simulink model "momentumBasedFlight"  (R2023b)
settings: Solver=VariableStepAuto  StartTime=0.0  StopTime=Config.simulationTime  RelTol=1e-3
InitFcn:
  | cd(fileparts(which(bdroot)));
  | initMomentumBasedFlight;
StopFcn:
  | cd(fileparts(which(bdroot)));
  | stopMomentumBasedFlight;
undefined symbols (not defined in the file or in its folder): aero_config, biasVectorConstraint_feet, Config, confVisualizer, ConstraintMatrix_feet, DiscIntNeverNeededParam, frameNames, Frames, jets_config, robot_config
libraries: WBToolboxLibrary x82, momentum_flight_control_v1 x1, deeplib x1, mwbs_robotDynamicsWithContacts_lib x1
(part 2 of 3)

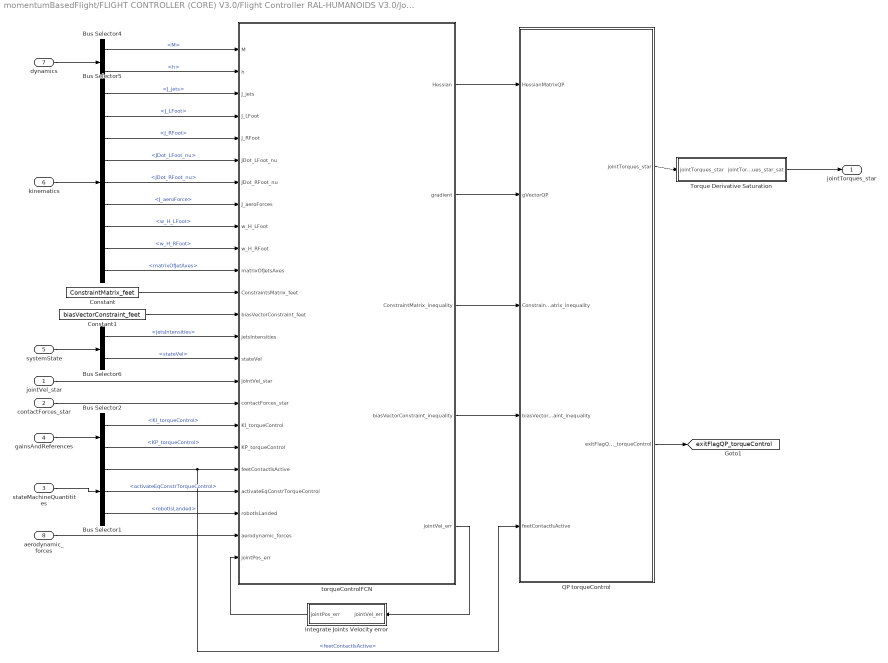
== system momentumBasedFlight/FLIGHT CONTROLLER (CORE) V3.0/Flight Controller RAL-HUMANOIDS V3.0/Joint Torque Control for Flying ==
  jointVel_star : Inport
  contactForces_star : Inport  Port=2
  stateMachineQuantitites : Inport  Port=3
  gainsAndReferences : Inport  Port=4
  systemState : Inport  Port=5
  kinematics : Inport  Port=6
  dynamics : Inport  Port=7
  aerodynamic_forces : Inport  Port=8
  Bus Selector1 : BusSelector  OutputSignals=feetContactIsActive,activateEqConstrTorqueControl,robotIsLanded
  Bus Selector2 : BusSelector  OutputSignals=KI_torqueControl,KP_torqueControl
  Bus Selector4 : BusSelector  OutputSignals=M,h
  Bus Selector5 : BusSelector  OutputSignals=J_jets,J_LFoot,J_RFoot,JDot_LFoot_nu,JDot_RFoot_nu,J_aeroForce,w_H_LFoot,w_H_RFoot,matrixOfJetAxes
  Bus Selector6 : BusSelector  OutputSignals=jetsIntensities,stateVel
  Constant : Constant  Value=ConstraintMatrix_feet
  Constant1 : Constant  Value=biasVectorConstraint_feet
  Integrate Joints Velocity error : Subsystem
  QP torqueControl : Subsystem
  Torque Derivative Saturation : Subsystem
  torqueControlFCN : MATLAB Function  TreatAsAtomicUnit=on
  jointTorques_star : Outport  VectorParamsAs1DForOutWhenUnconnected=off
  tag scope: exitFlagQP_torqueControl=global
  wires:
  Torque Derivative Saturation/1(jointTorques_star_sat) -> jointTorques_star/1
  Bus Selector1/2 -> torqueControlFCN/21(activateEqConstrTorqueControl)  "<activateEqConstrTorqueControl>"
  Bus Selector1/3 -> torqueControlFCN/22(robotIsLanded)  "<robotIsLanded>"
  torqueControlFCN/5(jointVel_err) -> Integrate Joints Velocity error/1(jointVel_err)
  Integrate Joints Velocity error/1(jointPos_err) -> torqueControlFCN/24(jointPos_err)
  Bus Selector5/9 -> torqueControlFCN/11(matrixOfJetsAxes)  "<matrixOfJetAxes>"
  jointVel_star/1 -> torqueControlFCN/16(jointVel_star)
  torqueControlFCN/4(biasVectorConstraint_inequality) -> QP torqueControl/4(biasVectorConstraint_inequality)
  torqueControlFCN/3(ConstraintMatrix_inequality) -> QP torqueControl/3(ConstraintMatrix_inequality)
  torqueControlFCN/2(gradient) -> QP torqueControl/2(gVectorQP)
  torqueControlFCN/1(Hessian) -> QP torqueControl/1(HessianMatrixQP)
  Bus Selector2/2 -> torqueControlFCN/19(KP_torqueControl)  "<KP_torqueControl>"
  Bus Selector2/1 -> torqueControlFCN/18(KI_torqueControl)  "<KI_torqueControl>"
  gainsAndReferences/1 -> Bus Selector2/1
  Bus Selector1/1 -> QP torqueControl/5(feetContactIsActive), torqueControlFCN/20(feetContactIsActive)  "<feetContactIsActive>"
  stateMachineQuantitites/1 -> Bus Selector1/1
  Bus Selector6/1 -> torqueControlFCN/14(jetsIntensities)  "<jetsIntensities>"
  QP torqueControl/2(exitFlagQP_torqueControl) -> [exitFlagQP_torqueControl]
  QP torqueControl/1(jointTorques_star) -> Torque Derivative Saturation/1(jointTorques_star)
  contactForces_star/1 -> torqueControlFCN/17(contactForces_star)
  Constant/1 -> torqueControlFCN/12(ConstraintsMatrix_feet)
  Constant1/1 -> torqueControlFCN/13(biasVectorConstraint_feet)
  Bus Selector5/8 -> torqueControlFCN/10(w_H_RFoot)  "<w_H_RFoot>"
  Bus Selector5/7 -> torqueControlFCN/9(w_H_LFoot)  "<w_H_LFoot>"
  Bus Selector5/5 -> torqueControlFCN/7(JDot_RFoot_nu)  "<JDot_RFoot_nu>"
  Bus Selector5/4 -> torqueControlFCN/6(JDot_LFoot_nu)  "<JDot_LFoot_nu>"
  Bus Selector5/3 -> torqueControlFCN/5(J_RFoot)  "<J_RFoot>"
  Bus Selector5/2 -> torqueControlFCN/4(J_LFoot)  "<J_LFoot>"
  Bus Selector5/1 -> torqueControlFCN/3(J_jets)  "<J_jets>"
  Bus Selector4/2 -> torqueControlFCN/2(h)  "<h>"
  Bus Selector4/1 -> torqueControlFCN/1(M)  "<M>"
  kinematics/1 -> Bus Selector5/1
  systemState/1 -> Bus Selector6/1
  dynamics/1 -> Bus Selector4/1
  Bus Selector6/2 -> torqueControlFCN/15(stateVel)  "<stateVel>"
  Bus Selector5/6 -> torqueControlFCN/8(J_aeroForces)  "<J_aeroForce>"
  aerodynamic_forces/1 -> torqueControlFCN/23(aerodynamic_forces)

== system momentumBasedFlight/FLIGHT CONTROLLER (CORE) V3.0/Flight Controller RAL-HUMANOIDS V3.0/Momentum Control for Flying ==
  stateMachineQuantitites : Inport
  gainsAndReferences : Inport  Port=2
  systemState : Inport  Port=3
  kinematics : Inport  Port=4
  dynamics : Inport  Port=5
  aerodynamic_forces : Inport  Port=6
  Momentum Control : Subsystem
  QP Solver and Integrate Contact Forces Derivative : Subsystem
  jointVel_star : Outport  VectorParamsAs1DForOutWhenUnconnected=off
  contactForces_star : Outport  Port=2  VectorParamsAs1DForOutWhenUnconnected=off
  jetsIntensitiesDot_star : Outport  Port=3  VectorParamsAs1DForOutWhenUnconnected=off
  wires:
  QP Solver and Integrate Contact Forces Derivative/3(jointVel_star) -> jointVel_star/1
  QP Solver and Integrate Contact Forces Derivative/1(contactForces_star) -> Momentum Control/1(contactForces_hat), contactForces_star/1  "WARNING! estimated contact forces are assumed to be coincident with contactForces_star"
  Momentum Control/4(uppeBoundQP) -> QP Solver and Integrate Contact Forces Derivative/4(upperBoundQP)
  Momentum Control/3(lowerBoundQP) -> QP Solver and Integrate Contact Forces Derivative/3(lowerBoundQP)
  Momentum Control/2(gVectorQP) -> QP Solver and Integrate Contact Forces Derivative/2(gVectorQP)
  Momentum Control/1(HessianMatrixQP) -> QP Solver and Integrate Contact Forces Derivative/1(HessianMatrixQP)
  stateMachineQuantitites/1 -> QP Solver and Integrate Contact Forces Derivative/5(stateMachineQuantities), Momentum Control/6(stateMachineQuantitites)
  gainsAndReferences/1 -> Momentum Control/5(gainsAndReferences)
  dynamics/1 -> Momentum Control/4(dynamics)
  kinematics/1 -> Momentum Control/3(kinematics)
  systemState/1 -> QP Solver and Integrate Contact Forces Derivative/6(systemState), Momentum Control/2(systemState)
  QP Solver and Integrate Contact Forces Derivative/2(jetsIntensitiesDot_star) -> jetsIntensitiesDot_star/1
  aerodynamic_forces/1 -> Momentum Control/7(aerodynamic_forces)

== system momentumBasedFlight/FLIGHT CONTROLLER (CORE) V3.0/Get System State/Change Contact Forces Representation ==
  jointPos : Inport
  w_H_b : Inport  Port=2
  contactForces_WBD : Inport  Port=3
  Change Contact Forces Representation : MATLAB Function  TreatAsAtomicUnit=on
  "CoM6D -> CoMXYZ1" : Selector  NumberOfDimensions=2  InputPortWidth=7  IndexOptions=Index vector (dialog),Index vector (dialog)  Indices=[1 2 3],[1 2 3]  OutputSizes=1,1
  "CoM6D -> CoMXYZ3" : Selector  NumberOfDimensions=2  InputPortWidth=7  IndexOptions=Index vector (dialog),Index vector (dialog)  Indices=[1 2 3],[1 2 3]  OutputSizes=1,1
  LFoot Pose : WBToolboxLibrary/Model/Kinematics/ForwardKinematics  frameName=Frames.LFOOT_FRAME
      settings: SourceProductName=WholeBodyToolbox
  Mux : Mux  Inputs=2
  RFoot Pose : WBToolboxLibrary/Model/Kinematics/ForwardKinematics  frameName=Frames.RFOOT_FRAME
      settings: SourceProductName=WholeBodyToolbox
  contactForces : Outport  VectorParamsAs1DForOutWhenUnconnected=off
  tag scope: wrench_LFoot=global, wrench_RFoot=global
  wires:
  contactForces_WBD/1 -> Change Contact Forces Representation/1(contactForces_WBD)
  RFoot Pose/1 -> "CoM6D -> CoMXYZ3"/1
  "CoM6D -> CoMXYZ3"/1 -> Change Contact Forces Representation/3(w_R_r_sole)
  LFoot Pose/1 -> "CoM6D -> CoMXYZ1"/1
  "CoM6D -> CoMXYZ1"/1 -> Change Contact Forces Representation/2(w_R_l_sole)
  w_H_b/1 -> LFoot Pose/1, RFoot Pose/1
  jointPos/1 -> LFoot Pose/2, RFoot Pose/2
  Change Contact Forces Representation/1(mixed_f_l_sole) -> [wrench_LFoot], Mux/1
  Change Contact Forces Representation/2(mixed_f_r_sole) -> [wrench_RFoot], Mux/2
  Mux/1 -> contactForces/1

== system momentumBasedFlight/FLIGHT CONTROLLER (CORE) V3.0/Jets Control/Feedback linearization ==
  jetState : Inport
  jetDerivatives_des : Inport  Port=2
  Bus Selector : BusSelector  OutputSignals=jetIntensitiesFiltered,jetDerivativesEst
  Discrete-Time Integrator : DiscreteIntegrator  SampleTime=Config.tStep  ICPrevOutput=DiscIntNeverNeededParam  ICPrevScaledInput=DiscIntNeverNeededParam
  Error : Scope
  MATLAB Function : MATLAB Function  TreatAsAtomicUnit=on
  jetDerivatives : Scope  NumInputPorts=3
  throttle : Outport  VectorParamsAs1DForOutWhenUnconnected=off
  wires:
  Bus Selector/1 -> MATLAB Function/1(jets)  "<jetIntensitiesFiltered>"
  MATLAB Function/1(throttle) -> jetDerivatives/1, throttle/1  "throttle"
  jetState/1 -> Bus Selector/1
  MATLAB Function/2(error) -> Error/1, Discrete-Time Integrator/1  "error"
  Bus Selector/2 -> jetDerivatives/3, MATLAB Function/2(jets_dot)  "<jetDerivativesEst>"
  Discrete-Time Integrator/1 -> MATLAB Function/4(integral_err)
  jetDerivatives_des/1 -> MATLAB Function/3(jets_dot_des), jetDerivatives/2

== system momentumBasedFlight/FLIGHT CONTROLLER (CORE) V3.0/Jets Control/extendedKalmanFilter4jets ==
  "jetsIntensityMeasured " : Inport
  "jetsThrottle " : Inport  Port=2
  Bus Creator : BusCreator  Inputs=2
  Demux : Demux
  Demux1 : Demux
  EKF_jet1 : Subsystem
  EKF_jet2 : Subsystem
  EKF_jet3 : Subsystem
  EKF_jet4 : Subsystem
  Mux : Mux
  Mux1 : Mux
  jetsState : Outport
  wires:
  Demux/1 -> EKF_jet1/1(input)
  Demux/2 -> EKF_jet2/1(input)
  Demux/3 -> EKF_jet3/1(input)
  Demux/4 -> EKF_jet4/1(input)
  Demux1/1 -> EKF_jet1/2(jetIntensityMeasurement)
  Demux1/2 -> EKF_jet2/2(jetIntensityMeasurement)
  Demux1/3 -> EKF_jet3/2(jetIntensityMeasurement)
  Demux1/4 -> EKF_jet4/2(jetIntensityMeasurement)
  EKF_jet2/1(jetIntensityFiltered) -> Mux/2
  EKF_jet1/1(jetIntensityFiltered) -> Mux/1
  EKF_jet3/1(jetIntensityFiltered) -> Mux/3
  EKF_jet4/1(jetIntensityFiltered) -> Mux/4
  EKF_jet1/2(jetDerivativeEstimated) -> Mux1/1
  EKF_jet2/2(jetDerivativeEstimated) -> Mux1/2
  EKF_jet3/2(jetDerivativeEstimated) -> Mux1/3
  EKF_jet4/2(jetDerivativeEstimated) -> Mux1/4
  "jetsThrottle "/1 -> Demux/1
  "jetsIntensityMeasured "/1 -> Demux1/1
  Mux/1 -> Bus Creator/1  "jetIntensitiesFiltered"
  Mux1/1 -> Bus Creator/2  "jetDerivativesEst"
  Bus Creator/1 -> jetsState/1

== system momentumBasedFlight/Visualizer/Task and Base Frame Kinematics/Combine Rotations ==
  roll : Inport
  pitch : Inport  Port=2
  yaw : Inport  Port=3
  roll_des : Inport  Port=4
  pitch_des : Inport  Port=5
  yaw_des : Inport  Port=6
  Mux : Mux  Inputs=2
  Mux1 : Mux  Inputs=2
  Mux2 : Mux  Inputs=2
  Task rotation combined : Scope  NumInputPorts=3
  wires:
  yaw_des/1 -> Mux2/2
  pitch_des/1 -> Mux1/2
  pitch/1 -> Mux1/1
  roll/1 -> Mux/1
  yaw/1 -> Mux2/1
  roll_des/1 -> Mux/2
  Mux2/1 -> Task rotation combined/3
  Mux1/1 -> Task rotation combined/2
  Mux/1 -> Task rotation combined/1

== system momentumBasedFlight/iRonCub/Forward Dynamics/AerodyNNamics ==
  state : Inport
  windSpeed : Inport  Port=2
  Bus Selector2 : BusSelector  OutputSignals=w_H_b,basePose_dot,joints_position
  Compute AerodyNNamics Inputs : MATLAB Function  TreatAsAtomicUnit=on
  Rotate Output from aerodynamic to world frame : MATLAB Function  TreatAsAtomicUnit=on
  aerodyNNamics : deeplib/Predict  Network=Network from MAT-file  NetworkFunction=squeezenet  NetworkFilePath=C:\Users\apaolino\code\element_aerodynamics-control\software\aerodynamic-flight-controllers\whole-body-aerodynamics-flight\src\aeroNet\aeroNet.mat  MiniBatchSize=1  InputDataFormats={ 'windDirection', 'CB'; 'jointPos', 'CB' }  Predictions=on  Activations={}  ForceInterpretedSim=off  EnableDLNetwork=on
  aerodynamicForceAreas : Outport
  wires:
  Bus Selector2/1 -> Rotate Output from aerodynamic to world frame/1(w_H_b), Compute AerodyNNamics Inputs/1(w_H_b)  "<w_H_b>"
  Bus Selector2/2 -> Compute AerodyNNamics Inputs/2(base_velocity)  "<basePose_dot>"
  Bus Selector2/3 -> Compute AerodyNNamics Inputs/3(joints_position)  "<joints_position>"
  state/1 -> Bus Selector2/1
  windSpeed/1 -> Compute AerodyNNamics Inputs/4(windSpeed)
  Compute AerodyNNamics Inputs/1(b_relWindDir) -> aerodyNNamics/1
  Rotate Output from aerodynamic to world frame/1(w_aerodynamicForceAreas) -> aerodynamicForceAreas/1
  Compute AerodyNNamics Inputs/2(jointPosDeg) -> aerodyNNamics/2
  aerodyNNamics/1 -> Rotate Output from aerodynamic to world frame/2(aerodynamicForceAreas)

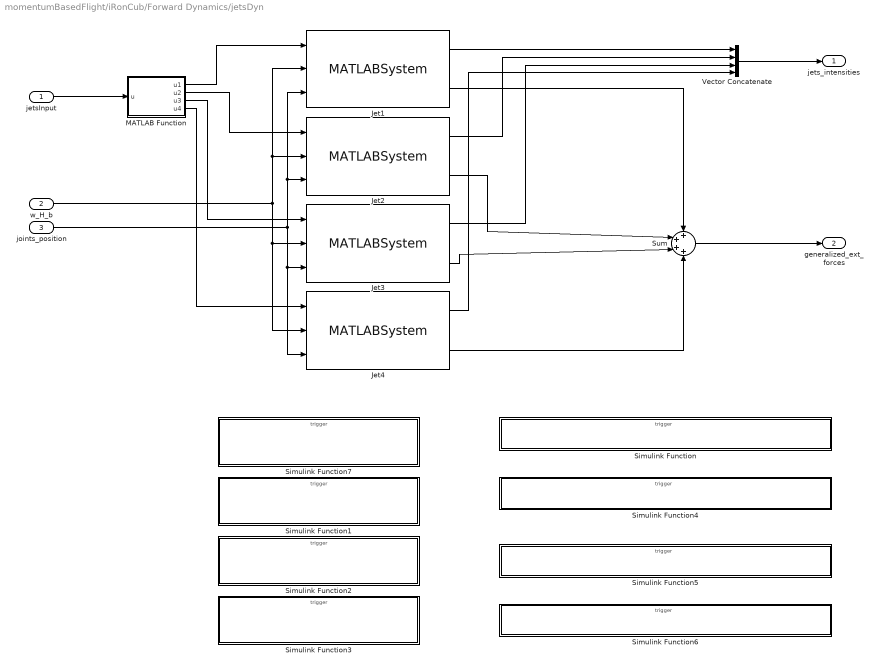
== system momentumBasedFlight/iRonCub/Forward Dynamics/jetsDyn ==
  jetsInput : Inport
  w_H_b : Inport  Port=2
  joints_position : Inport  Port=3
  Jet1 : MATLABSystem  System=jetDyn  jets_config=jets_config  tStep=Config.tStep  idx=1  SimulateUsing=Code generation
      mask Type: jetDyn
      mask Display:
      | disp('jetDyn');
      | port_label('input',1,'jet_input');
      | port_label('input',2,'basePose');
      | port_label('input',3,'jointPosition');
      | port_label('output',1,'jet_intensitiy');
      | port_label('output',2,'generalized_jet_wrench');
  Jet2 : MATLABSystem  System=jetDyn  jets_config=jets_config  tStep=Config.tStep  idx=2  SimulateUsing=Code generation
      mask Type: jetDyn
      mask Display:
      | disp('jetDyn');
      | port_label('input',1,'jet_input');
      | port_label('input',2,'basePose');
      | port_label('input',3,'jointPosition');
      | port_label('output',1,'jet_intensitiy');
      | port_label('output',2,'generalized_jet_wrench');
  Jet3 : MATLABSystem  System=jetDyn  jets_config=jets_config  tStep=Config.tStep  idx=3  SimulateUsing=Code generation
      mask Type: jetDyn
      mask Display:
      | disp('jetDyn');
      | port_label('input',1,'jet_input');
      | port_label('input',2,'basePose');
      | port_label('input',3,'jointPosition');
      | port_label('output',1,'jet_intensitiy');
      | port_label('output',2,'generalized_jet_wrench');
  Jet4 : MATLABSystem  System=jetDyn  jets_config=jets_config  tStep=Config.tStep  idx=4  SimulateUsing=Code generation
      mask Type: jetDyn
      mask Display:
      | disp('jetDyn');
      | port_label('input',1,'jet_input');
      | port_label('input',2,'basePose');
      | port_label('input',3,'jointPosition');
      | port_label('output',1,'jet_intensitiy');
      | port_label('output',2,'generalized_jet_wrench');
  MATLAB Function : MATLAB Function  TreatAsAtomicUnit=on
  Simulink Function : Subsystem  AncestorBlock=robotDynamicsWithContacts_lib/RobotDynWithContacts/Simulink Function  TreatAsAtomicUnit=on
  Simulink Function1 : Subsystem  AncestorBlock=robotDynamicsWithContacts_lib/RobotDynWithContacts/Simulink Function7  TreatAsAtomicUnit=on
  Simulink Function2 : Subsystem  AncestorBlock=robotDynamicsWithContacts_lib/RobotDynWithContacts/Simulink Function7  TreatAsAtomicUnit=on
  Simulink Function3 : Subsystem  AncestorBlock=robotDynamicsWithContacts_lib/RobotDynWithContacts/Simulink Function7  TreatAsAtomicUnit=on
  Simulink Function4 : Subsystem  AncestorBlock=robotDynamicsWithContacts_lib/RobotDynWithContacts/Simulink Function  TreatAsAtomicUnit=on
  Simulink Function5 : Subsystem  AncestorBlock=robotDynamicsWithContacts_lib/RobotDynWithContacts/Simulink Function  TreatAsAtomicUnit=on
  Simulink Function6 : Subsystem  AncestorBlock=robotDynamicsWithContacts_lib/RobotDynWithContacts/Simulink Function  TreatAsAtomicUnit=on
  Simulink Function7 : Subsystem  AncestorBlock=robotDynamicsWithContacts_lib/RobotDynWithContacts/Simulink Function7  TreatAsAtomicUnit=on
  Sum : Sum  Inputs=++++
  Vector Concatenate : Concatenate  NumInputs=4
  jets_intensities : Outport
  generalized_ext_forces : Outport  Port=2
  wires:
  Jet1/1 -> Vector Concatenate/1
  w_H_b/1 -> Jet2/2, Jet1/2, Jet4/2, Jet3/2
  joints_position/1 -> Jet3/3, Jet4/3, Jet1/3, Jet2/3
  Jet2/1 -> Vector Concatenate/2
  Jet2/2 -> Sum/2
  Jet3/1 -> Vector Concatenate/3
  Jet3/2 -> Sum/3
  Jet4/1 -> Vector Concatenate/4
  Jet4/2 -> Sum/4
  jetsInput/1 -> MATLAB Function/1(u)
  MATLAB Function/1(u1) -> Jet1/1
  MATLAB Function/2(u2) -> Jet2/1
  MATLAB Function/3(u3) -> Jet3/1
  MATLAB Function/4(u4) -> Jet4/1
  Vector Concatenate/1 -> jets_intensities/1
  Jet1/2 -> Sum/1
  Sum/1 -> generalized_ext_forces/1

== system momentumBasedFlight/FLIGHT CONTROLLER (CORE) V3.0/Dynamics and Kinematics/Dynamic Quantities/Compute Centroidal Inertia ==
  M : Inport
  w_H_b : Inport  Port=2
  posCoM : Inport  Port=3
  Compute Centroidal Inertia : MATLAB Function  TreatAsAtomicUnit=on
  Selector : Selector  NumberOfDimensions=2  InputPortWidth=3  IndexOptions=Index vector (dialog),Index vector (dialog)  Indices=[1 2 3],4  OutputSizes=1,1
  w_I_c : Outport  VectorParamsAs1DForOutWhenUnconnected=off
  wires:
  Compute Centroidal Inertia/1(w_I_c) -> w_I_c/1
  posCoM/1 -> Compute Centroidal Inertia/2(posCoM)
  Selector/1 -> Compute Centroidal Inertia/3(posBase)
  w_H_b/1 -> Selector/1
  M/1 -> Compute Centroidal Inertia/1(M)

== system momentumBasedFlight/FLIGHT CONTROLLER (CORE) V3.0/Dynamics and Kinematics/Dynamic Quantities/Momentum and CentroidalMomentum Matrix ==
  w_H_b : Inport
  jointPos : Inport  Port=2
  w_baseTwist : Inport  Port=3
  jointVel : Inport  Port=4
  CentroidalMomentum : WBToolboxLibrary/Model/Dynamics/CentroidalMomentum
      settings: SourceProductName=WholeBodyToolbox
  CentroidalTotalMomentumMatrix : WBToolboxLibrary/Model/Jacobians/CentroidalTotalMomentumMatrix
      settings: SourceProductName=WholeBodyToolbox
  L : Outport  VectorParamsAs1DForOutWhenUnconnected=off
  CMM : Outport  Port=2  VectorParamsAs1DForOutWhenUnconnected=off
  wires:
  CentroidalTotalMomentumMatrix/1 -> CMM/1
  jointVel/1 -> CentroidalMomentum/4
  jointPos/1 -> CentroidalMomentum/2, CentroidalTotalMomentumMatrix/2
  w_H_b/1 -> CentroidalMomentum/1, CentroidalTotalMomentumMatrix/1
  CentroidalMomentum/1 -> L/1
  w_baseTwist/1 -> CentroidalMomentum/3

== system momentumBasedFlight/FLIGHT CONTROLLER (CORE) V3.0/Dynamics and Kinematics/Kinematic Quantities/Compute Aerodynamic Forces Arms ==
  posCoM : Inport
  w_H_b : Inport  Port=2
  jointPos : Inport  Port=3
  Matrix Concatenate : Concatenate  NumInputs=13  Mode=Multidimensional array  ConcatenateDimension=2
  Pose Link 1 : WBToolboxLibrary/Model/Kinematics/ForwardKinematics  frameName=frameNames{1}
      settings: SourceProductName=WholeBodyToolbox
  Pose Link 10 : WBToolboxLibrary/Model/Kinematics/ForwardKinematics  frameName=frameNames{10}
      settings: SourceProductName=WholeBodyToolbox
  Pose Link 11 : WBToolboxLibrary/Model/Kinematics/ForwardKinematics  frameName=frameNames{11}
      settings: SourceProductName=WholeBodyToolbox
  Pose Link 12 : WBToolboxLibrary/Model/Kinematics/ForwardKinematics  frameName=frameNames{12}
      settings: SourceProductName=WholeBodyToolbox
  Pose Link 13 : WBToolboxLibrary/Model/Kinematics/ForwardKinematics  frameName=frameNames{13}
      settings: SourceProductName=WholeBodyToolbox
  Pose Link 2 : WBToolboxLibrary/Model/Kinematics/ForwardKinematics  frameName=frameNames{2}
      settings: SourceProductName=WholeBodyToolbox
  Pose Link 3 : WBToolboxLibrary/Model/Kinematics/ForwardKinematics  frameName=frameNames{3}
      settings: SourceProductName=WholeBodyToolbox
  Pose Link 4 : WBToolboxLibrary/Model/Kinematics/ForwardKinematics  frameName=frameNames{4}
      settings: SourceProductName=WholeBodyToolbox
  Pose Link 5 : WBToolboxLibrary/Model/Kinematics/ForwardKinematics  frameName=frameNames{5}
      settings: SourceProductName=WholeBodyToolbox
  Pose Link 6 : WBToolboxLibrary/Model/Kinematics/ForwardKinematics  frameName=frameNames{6}
      settings: SourceProductName=WholeBodyToolbox
  Pose Link 7 : WBToolboxLibrary/Model/Kinematics/ForwardKinematics  frameName=frameNames{7}
      settings: SourceProductName=WholeBodyToolbox
  Pose Link 8 : WBToolboxLibrary/Model/Kinematics/ForwardKinematics  frameName=frameNames{8}
      settings: SourceProductName=WholeBodyToolbox
  Pose Link 9 : WBToolboxLibrary/Model/Kinematics/ForwardKinematics  frameName=frameNames{9}
      settings: SourceProductName=WholeBodyToolbox
  Thrust Axes and Arms : MATLAB Function  TreatAsAtomicUnit=on
  matrixOfAeroArms : Outport  VectorParamsAs1DForOutWhenUnconnected=off
  wires:
  posCoM/1 -> Thrust Axes and Arms/2(posCoM)
  w_H_b/1 -> Pose Link 1/1, Pose Link 4/1, Pose Link 5/1, Pose Link 6/1, Pose Link 7/1, Pose Link 9/1, Pose Link 10/1, Pose Link 11/1, Pose Link 12/1, Pose Link 13/1, Pose Link 8/1, Pose Link 3/1, Pose Link 2/1
  Thrust Axes and Arms/1(matrixOfAeroArms) -> matrixOfAeroArms/1
  jointPos/1 -> Pose Link 13/2, Pose Link 12/2, Pose Link 11/2, Pose Link 10/2, Pose Link 9/2, Pose Link 8/2, Pose Link 7/2, Pose Link 6/2, Pose Link 5/2, Pose Link 4/2, Pose Link 3/2, Pose Link 2/2, Pose Link 1/2
  Matrix Concatenate/1 -> Thrust Axes and Arms/1(w_H_LinkFrames)
  Pose Link 13/1 -> Matrix Concatenate/13
  Pose Link 12/1 -> Matrix Concatenate/12
  Pose Link 11/1 -> Matrix Concatenate/11
  Pose Link 10/1 -> Matrix Concatenate/10
  Pose Link 9/1 -> Matrix Concatenate/9
  Pose Link 8/1 -> Matrix Concatenate/8
  Pose Link 7/1 -> Matrix Concatenate/7
  Pose Link 6/1 -> Matrix Concatenate/6
  Pose Link 5/1 -> Matrix Concatenate/5
  Pose Link 4/1 -> Matrix Concatenate/4
  Pose Link 3/1 -> Matrix Concatenate/3
  Pose Link 2/1 -> Matrix Concatenate/2
  Pose Link 1/1 -> Matrix Concatenate/1

== system momentumBasedFlight/FLIGHT CONTROLLER (CORE) V3.0/Dynamics and Kinematics/Kinematic Quantities/Compute Aerodynamic Forces Homogeneous Transform ==
  posCoM : Inport
  w_H_b : Inport  Port=2
  jointPos : Inport  Port=3
  Aero Transforms : MATLAB Function  TreatAsAtomicUnit=on
  Matrix Concatenate : Concatenate  NumInputs=13  Mode=Multidimensional array  ConcatenateDimension=2
  Pose Link 1 : WBToolboxLibrary/Model/Kinematics/ForwardKinematics  frameName=frameNames{1}
      settings: SourceProductName=WholeBodyToolbox
  Pose Link 10 : WBToolboxLibrary/Model/Kinematics/ForwardKinematics  frameName=frameNames{10}
      settings: SourceProductName=WholeBodyToolbox
  Pose Link 11 : WBToolboxLibrary/Model/Kinematics/ForwardKinematics  frameName=frameNames{11}
      settings: SourceProductName=WholeBodyToolbox
  Pose Link 12 : WBToolboxLibrary/Model/Kinematics/ForwardKinematics  frameName=frameNames{12}
      settings: SourceProductName=WholeBodyToolbox
  Pose Link 13 : WBToolboxLibrary/Model/Kinematics/ForwardKinematics  frameName=frameNames{13}
      settings: SourceProductName=WholeBodyToolbox
  Pose Link 2 : WBToolboxLibrary/Model/Kinematics/ForwardKinematics  frameName=frameNames{2}
      settings: SourceProductName=WholeBodyToolbox
  Pose Link 3 : WBToolboxLibrary/Model/Kinematics/ForwardKinematics  frameName=frameNames{3}
      settings: SourceProductName=WholeBodyToolbox
  Pose Link 4 : WBToolboxLibrary/Model/Kinematics/ForwardKinematics  frameName=frameNames{4}
      settings: SourceProductName=WholeBodyToolbox
  Pose Link 5 : WBToolboxLibrary/Model/Kinematics/ForwardKinematics  frameName=frameNames{5}
      settings: SourceProductName=WholeBodyToolbox
  Pose Link 6 : WBToolboxLibrary/Model/Kinematics/ForwardKinematics  frameName=frameNames{6}
      settings: SourceProductName=WholeBodyToolbox
  Pose Link 7 : WBToolboxLibrary/Model/Kinematics/ForwardKinematics  frameName=frameNames{7}
      settings: SourceProductName=WholeBodyToolbox
  Pose Link 8 : WBToolboxLibrary/Model/Kinematics/ForwardKinematics  frameName=frameNames{8}
      settings: SourceProductName=WholeBodyToolbox
  Pose Link 9 : WBToolboxLibrary/Model/Kinematics/ForwardKinematics  frameName=frameNames{9}
      settings: SourceProductName=WholeBodyToolbox
  matrixOfCoMTransform : Outport  VectorParamsAs1DForOutWhenUnconnected=off
  wires:
  posCoM/1 -> Aero Transforms/2(posCoM)
  w_H_b/1 -> Pose Link 1/1, Pose Link 4/1, Pose Link 5/1, Pose Link 6/1, Pose Link 7/1, Pose Link 9/1, Pose Link 10/1, Pose Link 11/1, Pose Link 12/1, Pose Link 13/1, Pose Link 8/1, Pose Link 3/1, Pose Link 2/1
  Aero Transforms/1(matrixOfLinkCoMTransform) -> matrixOfCoMTransform/1
  jointPos/1 -> Pose Link 13/2, Pose Link 12/2, Pose Link 11/2, Pose Link 10/2, Pose Link 9/2, Pose Link 8/2, Pose Link 7/2, Pose Link 6/2, Pose Link 5/2, Pose Link 4/2, Pose Link 3/2, Pose Link 2/2, Pose Link 1/2
  Matrix Concatenate/1 -> Aero Transforms/1(w_H_LinkFrames)
  Pose Link 13/1 -> Matrix Concatenate/13
  Pose Link 12/1 -> Matrix Concatenate/12
  Pose Link 11/1 -> Matrix Concatenate/11
  Pose Link 10/1 -> Matrix Concatenate/10
  Pose Link 9/1 -> Matrix Concatenate/9
  Pose Link 8/1 -> Matrix Concatenate/8
  Pose Link 7/1 -> Matrix Concatenate/7
  Pose Link 6/1 -> Matrix Concatenate/6
  Pose Link 5/1 -> Matrix Concatenate/5
  Pose Link 4/1 -> Matrix Concatenate/4
  Pose Link 3/1 -> Matrix Concatenate/3
  Pose Link 2/1 -> Matrix Concatenate/2
  Pose Link 1/1 -> Matrix Concatenate/1

== system momentumBasedFlight/FLIGHT CONTROLLER (CORE) V3.0/Dynamics and Kinematics/Kinematic Quantities/Compute Aerodynamic Forces Jacobians ==
  w_H_b : Inport
  jointPos : Inport  Port=2
  Jacobian Link frame 1 : WBToolboxLibrary/Model/Jacobians/Jacobian  frameName=frameNames{1}
      settings: SourceProductName=WholeBodyToolbox
  Jacobian Link frame 10 : WBToolboxLibrary/Model/Jacobians/Jacobian  frameName=frameNames{10}
      settings: SourceProductName=WholeBodyToolbox
  Jacobian Link frame 11 : WBToolboxLibrary/Model/Jacobians/Jacobian  frameName=frameNames{11}
      settings: SourceProductName=WholeBodyToolbox
  Jacobian Link frame 12 : WBToolboxLibrary/Model/Jacobians/Jacobian  frameName=frameNames{12}
      settings: SourceProductName=WholeBodyToolbox
  Jacobian Link frame 13 : WBToolboxLibrary/Model/Jacobians/Jacobian  frameName=frameNames{13}
      settings: SourceProductName=WholeBodyToolbox
  Jacobian Link frame 2 : WBToolboxLibrary/Model/Jacobians/Jacobian  frameName=frameNames{2}
      settings: SourceProductName=WholeBodyToolbox
  Jacobian Link frame 3 : WBToolboxLibrary/Model/Jacobians/Jacobian  frameName=frameNames{3}
      settings: SourceProductName=WholeBodyToolbox
  Jacobian Link frame 4 : WBToolboxLibrary/Model/Jacobians/Jacobian  frameName=frameNames{4}
      settings: SourceProductName=WholeBodyToolbox
  Jacobian Link frame 5 : WBToolboxLibrary/Model/Jacobians/Jacobian  frameName=frameNames{5}
      settings: SourceProductName=WholeBodyToolbox
  Jacobian Link frame 6 : WBToolboxLibrary/Model/Jacobians/Jacobian  frameName=frameNames{6}
      settings: SourceProductName=WholeBodyToolbox
  Jacobian Link frame 7 : WBToolboxLibrary/Model/Jacobians/Jacobian  frameName=frameNames{7}
      settings: SourceProductName=WholeBodyToolbox
  Jacobian Link frame 8 : WBToolboxLibrary/Model/Jacobians/Jacobian  frameName=frameNames{8}
      settings: SourceProductName=WholeBodyToolbox
  Jacobian Link frame 9 : WBToolboxLibrary/Model/Jacobians/Jacobian  frameName=frameNames{9}
      settings: SourceProductName=WholeBodyToolbox
  Matrix Concatenate : Concatenate  NumInputs=13  Mode=Multidimensional array
  compute matrix of link CoM Jacobians : MATLAB Function  TreatAsAtomicUnit=on
  J_aeroForces : Outport  VectorParamsAs1DForOutWhenUnconnected=off
  wires:
  w_H_b/1 -> Jacobian Link frame 1/1, Jacobian Link frame 2/1, Jacobian Link frame 3/1, Jacobian Link frame 4/1, Jacobian Link frame 6/1, Jacobian Link frame 7/1, Jacobian Link frame 8/1, Jacobian Link frame 9/1, Jacobian Link frame 10/1, Jacobian Link frame 11/1, Jacobian Link frame 13/1, Jacobian Link frame 12/1, Jacobian Link frame 5/1, compute matrix of link CoM Jacobians/1(w_H_b)
  jointPos/1 -> Jacobian Link frame 13/2, Jacobian Link frame 12/2, Jacobian Link frame 11/2, Jacobian Link frame 10/2, Jacobian Link frame 9/2, Jacobian Link frame 8/2, Jacobian Link frame 7/2, Jacobian Link frame 6/2, Jacobian Link frame 4/2, Jacobian Link frame 3/2, Jacobian Link frame 1/2, Jacobian Link frame 2/2, Jacobian Link frame 5/2
  Jacobian Link frame 1/1 -> Matrix Concatenate/1
  Jacobian Link frame 2/1 -> Matrix Concatenate/2
  Jacobian Link frame 3/1 -> Matrix Concatenate/3
  Jacobian Link frame 5/1 -> Matrix Concatenate/5
  Jacobian Link frame 4/1 -> Matrix Concatenate/4
  Jacobian Link frame 6/1 -> Matrix Concatenate/6
  Jacobian Link frame 7/1 -> Matrix Concatenate/7
  Jacobian Link frame 8/1 -> Matrix Concatenate/8
  Jacobian Link frame 9/1 -> Matrix Concatenate/9
  Jacobian Link frame 10/1 -> Matrix Concatenate/10
  Jacobian Link frame 11/1 -> Matrix Concatenate/11
  Jacobian Link frame 12/1 -> Matrix Concatenate/12
  Jacobian Link frame 13/1 -> Matrix Concatenate/13
  compute matrix of link CoM Jacobians/1(J_aeroForces) -> J_aeroForces/1
  Matrix Concatenate/1 -> compute matrix of link CoM Jacobians/2(linkFrameJacobians)

== system momentumBasedFlight/FLIGHT CONTROLLER (CORE) V3.0/Dynamics and Kinematics/Kinematic Quantities/Compute Thrusts Axes and Arms ==
  posCoM : Inport
  w_H_b : Inport  Port=2
  jointPos : Inport  Port=3
  Pose Jet 1 : WBToolboxLibrary/Model/Kinematics/ForwardKinematics  frameName=Frames.JET1_FRAME
      settings: SourceProductName=WholeBodyToolbox
  Pose Jet 2 : WBToolboxLibrary/Model/Kinematics/ForwardKinematics  frameName=Frames.JET2_FRAME
      settings: SourceProductName=WholeBodyToolbox
  Pose Jet 3 : WBToolboxLibrary/Model/Kinematics/ForwardKinematics  frameName=Frames.JET3_FRAME
      settings: SourceProductName=WholeBodyToolbox
  Pose Jet 4 : WBToolboxLibrary/Model/Kinematics/ForwardKinematics  frameName=Frames.JET4_FRAME
      settings: SourceProductName=WholeBodyToolbox
  Thrust Axes and Arms : MATLAB Function  TreatAsAtomicUnit=on
  matrixOfJetsAxes : Outport  VectorParamsAs1DForOutWhenUnconnected=off
  matrixOfJetsArms : Outport  Port=2  VectorParamsAs1DForOutWhenUnconnected=off
  wires:
  posCoM/1 -> Thrust Axes and Arms/5(posCoM)
  w_H_b/1 -> Pose Jet 1/1, Pose Jet 2/1, Pose Jet 3/1, Pose Jet 4/1
  Thrust Axes and Arms/2(matrixOfJetsArms) -> matrixOfJetsArms/1
  Thrust Axes and Arms/1(matrixOfJetsAxes) -> matrixOfJetsAxes/1
  Pose Jet 4/1 -> Thrust Axes and Arms/4(w_H_J4)
  Pose Jet 3/1 -> Thrust Axes and Arms/3(w_H_J3)
  Pose Jet 1/1 -> Thrust Axes and Arms/1(w_H_J1)
  jointPos/1 -> Pose Jet 4/2, Pose Jet 3/2, Pose Jet 2/2, Pose Jet 1/2
  Pose Jet 2/1 -> Thrust Axes and Arms/2(w_H_J2)

== system momentumBasedFlight/FLIGHT CONTROLLER (CORE) V3.0/Flight Controller RAL-HUMANOIDS V3.0/Joint Torque Control for Flying/Integrate Joints Velocity error ==
  jointVel_err : Inport
  Constant : Constant  Value=zeros(Config.N_DOF,1)
  Discrete-Time Integrator1 : DiscreteIntegrator  InitialConditionSource=external  InitialCondition=zeros(Config.N_DOF,1)  SampleTime=Config.tStep  UpperSaturationLimit=20  LowerSaturationLimit=-20  ICPrevOutput=DiscIntNeverNeededParam  ICPrevScaledInput=DiscIntNeverNeededParam
  jointPos_err : Outport  VectorParamsAs1DForOutWhenUnconnected=off
  tag scope: jointPos_err_integral=global
  wires:
  Constant/1 -> Discrete-Time Integrator1/2
  jointVel_err/1 -> Discrete-Time Integrator1/1
  Discrete-Time Integrator1/1 -> [jointPos_err_integral], jointPos_err/1

== system momentumBasedFlight/FLIGHT CONTROLLER (CORE) V3.0/Flight Controller RAL-HUMANOIDS V3.0/Joint Torque Control for Flying/QP torqueControl ==
  HessianMatrixQP : Inport
  gVectorQP : Inport  Port=2
  ConstraintMatrix_inequality : Inport  Port=3
  biasVectorConstraint_inequality : Inport  Port=4
  feetContactIsActive : Inport  Port=5
  Constant2 : Constant  Value=Config.sat.jointTorquesSaturation
  NOT : Logic  Operator=NOT  IconShape=distinctive  AllPortsSameDT=off  OutDataTypeStr=boolean
  Process QP Inputs Torque Control : MATLAB Function  TreatAsAtomicUnit=on
  QP torqueControl - balancing : Subsystem  TreatAsAtomicUnit=on
  QP torqueControl - flight : Subsystem  TreatAsAtomicUnit=on
  Select QP torqueControl Output : Subsystem
  jointTorques_star : Outport  VectorParamsAs1DForOutWhenUnconnected=off
  exitFlagQP_torqueControl : Outport  Port=2  VectorParamsAs1DForOutWhenUnconnected=off
  wires:
  Select QP torqueControl Output/1(jointTorques_star) -> jointTorques_star/1
  Select QP torqueControl Output/2(exitFlagQP_torqueControl) -> exitFlagQP_torqueControl/1
  QP torqueControl - flight/1(QPStatus_flight) -> Select QP torqueControl Output/4(QPStatus_flight)
  QP torqueControl - flight/2(QPOutput_flight) -> Select QP torqueControl Output/5(QPOutput_flight)
  QP torqueControl - balancing/2(QPOutput_balancing) -> Select QP torqueControl Output/2(QPOutput_balancing)
  QP torqueControl - balancing/1(QPStatus_balancing) -> Select QP torqueControl Output/1(QPStatus_balancing)
  Process QP Inputs Torque Control/1(H_balancing) -> QP torqueControl - balancing/1(H)
  Process QP Inputs Torque Control/2(g_balancing) -> QP torqueControl - balancing/2(g)
  Process QP Inputs Torque Control/3(ub_balancing) -> QP torqueControl - balancing/3(ub)
  Process QP Inputs Torque Control/4(lb_balancing) -> QP torqueControl - balancing/4(lb)
  Process QP Inputs Torque Control/5(Aeq_balancing) -> QP torqueControl - balancing/5(AEq)
  Process QP Inputs Torque Control/6(lbEq_balancing) -> QP torqueControl - balancing/6(lbEq)
  Process QP Inputs Torque Control/7(ubEq_balancing) -> QP torqueControl - balancing/7(ubEq)
  Process QP Inputs Torque Control/11(lb_flight) -> QP torqueControl - flight/4(lb)
  Process QP Inputs Torque Control/10(ub_flight) -> QP torqueControl - flight/3(ub)
  Process QP Inputs Torque Control/9(g_flight) -> QP torqueControl - flight/2(g)
  Process QP Inputs Torque Control/8(H_flight) -> QP torqueControl - flight/1(H)
  Constant2/1 -> Process QP Inputs Torque Control/5(jointTorquesSaturation)
  gVectorQP/1 -> Process QP Inputs Torque Control/2(gVectorQP)
  HessianMatrixQP/1 -> Process QP Inputs Torque Control/1(HessianMatrixQP)
  ConstraintMatrix_inequality/1 -> Process QP Inputs Torque Control/3(InequalityConstrMatrix)
  biasVectorConstraint_inequality/1 -> Process QP Inputs Torque Control/4(biasVectorInequalityConstr)
  NOT/1 -> QP torqueControl - flight/Enable
  feetContactIsActive/1 -> NOT/1, QP torqueControl - balancing/Enable, Select QP torqueControl Output/3(feetContactIsActive)

== system momentumBasedFlight/FLIGHT CONTROLLER (CORE) V3.0/Flight Controller RAL-HUMANOIDS V3.0/Joint Torque Control for Flying/Torque Derivative Saturation ==
  jointTorques_star : Inport
  Constant1 : Constant  Value=Config.tStep
  Constant2 : Constant  Value=Config.sat.jointTorquesDotMax
  Saturate Torque Derivative : MATLAB Function  TreatAsAtomicUnit=on
  "holder " : WBToolboxLibrary/Utilities/holder 
      settings: SourceProductName=WholeBodyToolbox
  jointTorques_star_sat : Outport  VectorParamsAs1DForOutWhenUnconnected=off
  wires:
  Constant2/1 -> Saturate Torque Derivative/4(uDotMax)
  Constant1/1 -> Saturate Torque Derivative/3(tStep)
  "holder "/1 -> Saturate Torque Derivative/2(u_0)
  Saturate Torque Derivative/1(uSat) -> jointTorques_star_sat/1
  jointTorques_star/1 -> Saturate Torque Derivative/1(u), "holder "/1

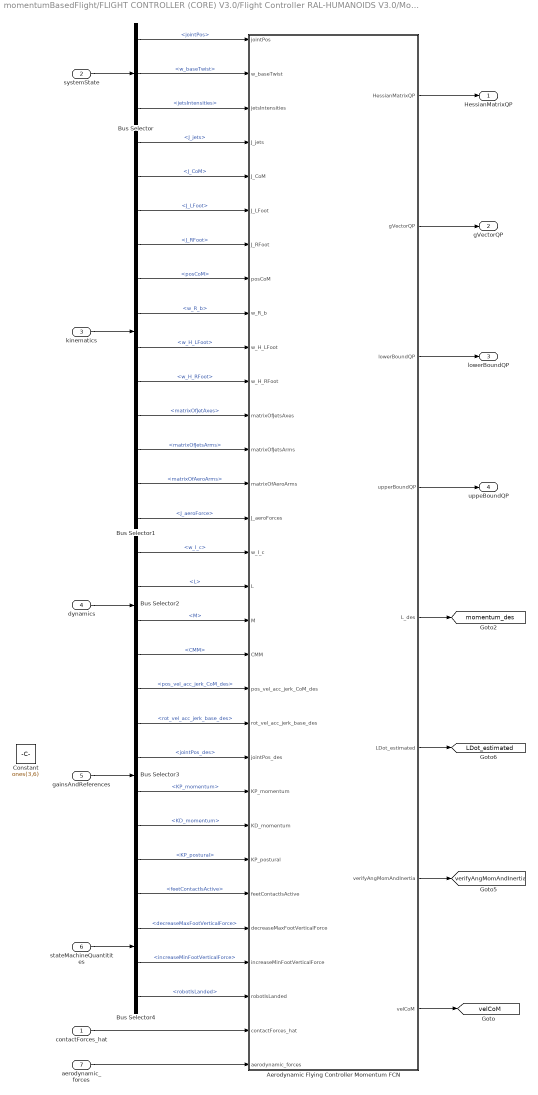
== system momentumBasedFlight/FLIGHT CONTROLLER (CORE) V3.0/Flight Controller RAL-HUMANOIDS V3.0/Momentum Control for Flying/Momentum Control ==
  contactForces_hat : Inport
  systemState : Inport  Port=2
  kinematics : Inport  Port=3
  dynamics : Inport  Port=4
  gainsAndReferences : Inport  Port=5
  stateMachineQuantitites : Inport  Port=6
  aerodynamic_forces : Inport  Port=7
  "Aerodynamic Flying Controller Momentum FCN " : MATLAB Function  TreatAsAtomicUnit=on
  Bus Selector : BusSelector  OutputSignals=jointPos,w_baseTwist,jetsIntensities
  Bus Selector1 : BusSelector  OutputSignals=J_jets,J_CoM,J_LFoot,J_RFoot,posCoM,w_R_b,w_H_LFoot,w_H_RFoot,matrixOfJetAxes,matrixOfJetsArms,matrixOfAeroArms,J_aeroForce
  Bus Selector2 : BusSelector  OutputSignals=w_I_c,L,M,CMM
  Bus Selector3 : BusSelector  OutputSignals=pos_vel_acc_jerk_CoM_des,rot_vel_acc_jerk_base_des,jointPos_des,KP_momentum,KD_momentum,KP_postural
  Bus Selector4 : BusSelector  OutputSignals=feetContactIsActive,decreaseMaxFootVerticalForce,increaseMinFootVerticalForce,robotIsLanded
  Constant : Constant  Value=ones(3,6)
  HessianMatrixQP : Outport  VectorParamsAs1DForOutWhenUnconnected=off
  gVectorQP : Outport  Port=2  VectorParamsAs1DForOutWhenUnconnected=off
  lowerBoundQP : Outport  Port=3  VectorParamsAs1DForOutWhenUnconnected=off
  uppeBoundQP : Outport  Port=4  VectorParamsAs1DForOutWhenUnconnected=off
  tag scope: LDot_estimated=global, momentum_des=global, velCoM=global, verifyAngMomAndInertia=global
  wires:
  "Aerodynamic Flying Controller Momentum FCN "/8(velCoM) -> [velCoM]
  contactForces_hat/1 -> "Aerodynamic Flying Controller Momentum FCN "/30(contactForces_hat)
  Bus Selector4/4 -> "Aerodynamic Flying Controller Momentum FCN "/29(robotIsLanded)  "<robotIsLanded>"
  Bus Selector4/3 -> "Aerodynamic Flying Controller Momentum FCN "/28(increaseMinFootVerticalForce)  "<increaseMinFootVerticalForce>"
  Bus Selector4/2 -> "Aerodynamic Flying Controller Momentum FCN "/27(decreaseMaxFootVerticalForce)  "<decreaseMaxFootVerticalForce>"
  Bus Selector2/1 -> "Aerodynamic Flying Controller Momentum FCN "/16(w_I_c)  "<w_I_c>"
  Bus Selector1/10 -> "Aerodynamic Flying Controller Momentum FCN "/13(matrixOfJetsArms)  "<matrixOfJetsArms>"
  Bus Selector1/9 -> "Aerodynamic Flying Controller Momentum FCN "/12(matrixOfJetsAxes)  "<matrixOfJetAxes>"
  Bus Selector3/1 -> "Aerodynamic Flying Controller Momentum FCN "/20(pos_vel_acc_jerk_CoM_des)  "<pos_vel_acc_jerk_CoM_des>"
  Bus Selector1/6 -> "Aerodynamic Flying Controller Momentum FCN "/9(w_R_b)  "<w_R_b>"
  Bus Selector1/5 -> "Aerodynamic Flying Controller Momentum FCN "/8(posCoM)  "<posCoM>"
  "Aerodynamic Flying Controller Momentum FCN "/5(L_des) -> [momentum_des]
  Bus Selector3/6 -> "Aerodynamic Flying Controller Momentum FCN "/25(KP_postural)  "<KP_postural>"
  Bus Selector2/2 -> "Aerodynamic Flying Controller Momentum FCN "/17(L)  "<L>"
  Bus Selector1/7 -> "Aerodynamic Flying Controller Momentum FCN "/10(w_H_LFoot)  "<w_H_LFoot>"
  Bus Selector3/5 -> "Aerodynamic Flying Controller Momentum FCN "/24(KD_momentum)  "<KD_momentum>"
  "Aerodynamic Flying Controller Momentum FCN "/6(LDot_estimated) -> [LDot_estimated]
  Bus Selector2/3 -> "Aerodynamic Flying Controller Momentum FCN "/18(M)  "<M>"
  Bus Selector2/4 -> "Aerodynamic Flying Controller Momentum FCN "/19(CMM)  "<CMM>"
  Bus Selector1/8 -> "Aerodynamic Flying Controller Momentum FCN "/11(w_H_RFoot)  "<w_H_RFoot>"
  Bus Selector1/4 -> "Aerodynamic Flying Controller Momentum FCN "/7(J_RFoot)  "<J_RFoot>"
  Bus Selector/3 -> "Aerodynamic Flying Controller Momentum FCN "/3(jetsIntensities)  "<jetsIntensities>"
  gainsAndReferences/1 -> Bus Selector3/1
  Bus Selector1/2 -> "Aerodynamic Flying Controller Momentum FCN "/5(J_CoM)  "<J_CoM>"
  dynamics/1 -> Bus Selector2/1
  Bus Selector3/4 -> "Aerodynamic Flying Controller Momentum FCN "/23(KP_momentum)  "<KP_momentum>"
  "Aerodynamic Flying Controller Momentum FCN "/3(lowerBoundQP) -> lowerBoundQP/1
  stateMachineQuantitites/1 -> Bus Selector4/1
  "Aerodynamic Flying Controller Momentum FCN "/7(verifyAngMomAndInertia) -> [verifyAngMomAndInertia]
  Bus Selector4/1 -> "Aerodynamic Flying Controller Momentum FCN "/26(feetContactIsActive)  "<feetContactIsActive>"
  "Aerodynamic Flying Controller Momentum FCN "/2(gVectorQP) -> gVectorQP/1
  "Aerodynamic Flying Controller Momentum FCN "/4(upperBoundQP) -> uppeBoundQP/1
  "Aerodynamic Flying Controller Momentum FCN "/1(HessianMatrixQP) -> HessianMatrixQP/1
  Bus Selector/2 -> "Aerodynamic Flying Controller Momentum FCN "/2(w_baseTwist)  "<w_baseTwist>"
  Bus Selector1/1 -> "Aerodynamic Flying Controller Momentum FCN "/4(J_jets)  "<J_jets>"
  Bus Selector/1 -> "Aerodynamic Flying Controller Momentum FCN "/1(jointPos)  "<jointPos>"
  kinematics/1 -> Bus Selector1/1
  Bus Selector1/3 -> "Aerodynamic Flying Controller Momentum FCN "/6(J_LFoot)  "<J_LFoot>"
  Bus Selector3/3 -> "Aerodynamic Flying Controller Momentum FCN "/22(jointPos_des)  "<jointPos_des>"
  systemState/1 -> Bus Selector/1
  Bus Selector3/2 -> "Aerodynamic Flying Controller Momentum FCN "/21(rot_vel_acc_jerk_base_des)  "<rot_vel_acc_jerk_base_des>"
  aerodynamic_forces/1 -> "Aerodynamic Flying Controller Momentum FCN "/31(aerodynamic_forces)
  Bus Selector1/11 -> "Aerodynamic Flying Controller Momentum FCN "/14(matrixOfAeroArms)  "<matrixOfAeroArms>"
  Bus Selector1/12 -> "Aerodynamic Flying Controller Momentum FCN "/15(J_aeroForces)  "<J_aeroForce>"

== system momentumBasedFlight/FLIGHT CONTROLLER (CORE) V3.0/Flight Controller RAL-HUMANOIDS V3.0/Momentum Control for Flying/QP Solver and Integrate Contact Forces Derivative ==
  HessianMatrixQP : Inport
  gVectorQP : Inport  Port=2
  lowerBoundQP : Inport  Port=3
  upperBoundQP : Inport  Port=4
  stateMachineQuantities : Inport  Port=5
  systemState : Inport  Port=6
  Bus Selector1 : BusSelector  OutputSignals=feetContactIsActive
  Bus Selector2 : BusSelector  OutputSignals=contactForces
  Integrate the Contact Forces Derivative : Subsystem
  QP momentumControl : Subsystem
  contactForces_star : Outport  VectorParamsAs1DForOutWhenUnconnected=off
  jetsIntensitiesDot_star : Outport  Port=2  VectorParamsAs1DForOutWhenUnconnected=off
  jointVel_star : Outport  Port=3  VectorParamsAs1DForOutWhenUnconnected=off
  tag scope: contactForces_star=global, exitFlagQP_momentumControl=global, jetsIntensitiesDot_star=global, jointVel_star=global
  wires:
  systemState/1 -> Bus Selector2/1
  Bus Selector2/1 -> Integrate the Contact Forces Derivative/2(contactForces)  "<contactForces>"
  Bus Selector1/1 -> Integrate the Contact Forces Derivative/3(feetContactIsActive), QP momentumControl/5(feetContactIsActive)  "<feetContactIsActive>"
  QP momentumControl/3(jointVel_star) -> jointVel_star/1, [jointVel_star]
  QP momentumControl/1(jetsIntensitiesDot_star) -> jetsIntensitiesDot_star/1, [jetsIntensitiesDot_star]
  HessianMatrixQP/1 -> QP momentumControl/1(HessianMatrixQP)
  stateMachineQuantities/1 -> Bus Selector1/1
  gVectorQP/1 -> QP momentumControl/2(gVectorQP)
  QP momentumControl/4(exitFlagQP_momentumControl) -> [exitFlagQP_momentumControl]
  upperBoundQP/1 -> QP momentumControl/4(upperBoundQP)
  lowerBoundQP/1 -> QP momentumControl/3(lowerBoundQP)
  Integrate the Contact Forces Derivative/1(contactForces_star) -> contactForces_star/1, [contactForces_star]
  QP momentumControl/2(contactForcesDot_star) -> Integrate the Contact Forces Derivative/1(contactForcesDot_star)

== system momentumBasedFlight/FLIGHT CONTROLLER (CORE) V3.0/Jets Control/extendedKalmanFilter4jets/EKF_jet1 ==
  input : Inport
  jetIntensityMeasurement : Inport  Port=2
  Constant : Constant  Value=[Config.initT, Config.initTdot]
  Constant1 : Constant  Value=Config.ekf.initP
  Discrete-Time Integrator1 : DiscreteIntegrator  InitialConditionSource=external  SampleTime=Config.tStep  ICPrevOutput=DiscIntNeverNeededParam  ICPrevScaledInput=DiscIntNeverNeededParam
  Discrete-Time Integrator2 : DiscreteIntegrator  InitialConditionSource=external  SampleTime=Config.tStep  ICPrevOutput=DiscIntNeverNeededParam  ICPrevScaledInput=DiscIntNeverNeededParam
  "EKF " : MATLAB Function  TreatAsAtomicUnit=on
  splitVector : MATLAB Function  TreatAsAtomicUnit=on
  jetIntensityFiltered : Outport  VectorParamsAs1DForOutWhenUnconnected=off
  jetDerivativeEstimated : Outport  Port=2  VectorParamsAs1DForOutWhenUnconnected=off
  wires:
  splitVector/2(x2) -> jetDerivativeEstimated/1
  splitVector/1(x1) -> jetIntensityFiltered/1
  Constant1/1 -> Discrete-Time Integrator2/2
  Discrete-Time Integrator2/1 -> "EKF "/4(P)
  jetIntensityMeasurement/1 -> "EKF "/3(measurement)
  Constant/1 -> Discrete-Time Integrator1/2
  Discrete-Time Integrator1/1 -> splitVector/1(x), "EKF "/1(x)
  input/1 -> "EKF "/2(input)
  "EKF "/1(xDot) -> Discrete-Time Integrator1/1
  "EKF "/2(Pdot) -> Discrete-Time Integrator2/1

== system momentumBasedFlight/FLIGHT CONTROLLER (CORE) V3.0/Jets Control/extendedKalmanFilter4jets/EKF_jet2 ==
  input : Inport
  jetIntensityMeasurement : Inport  Port=2
  Constant : Constant  Value=[Config.initT, Config.initTdot]
  Constant1 : Constant  Value=Config.ekf.initP
  Discrete-Time Integrator1 : DiscreteIntegrator  InitialConditionSource=external  SampleTime=Config.tStep  ICPrevOutput=DiscIntNeverNeededParam  ICPrevScaledInput=DiscIntNeverNeededParam
  Discrete-Time Integrator2 : DiscreteIntegrator  InitialConditionSource=external  SampleTime=Config.tStep  ICPrevOutput=DiscIntNeverNeededParam  ICPrevScaledInput=DiscIntNeverNeededParam
  "EKF " : MATLAB Function  TreatAsAtomicUnit=on
  splitVector : MATLAB Function  TreatAsAtomicUnit=on
  jetIntensityFiltered : Outport  VectorParamsAs1DForOutWhenUnconnected=off
  jetDerivativeEstimated : Outport  Port=2  VectorParamsAs1DForOutWhenUnconnected=off
  wires:
  "EKF "/2(Pdot) -> Discrete-Time Integrator2/1
  "EKF "/1(xDot) -> Discrete-Time Integrator1/1
  input/1 -> "EKF "/2(input)
  Discrete-Time Integrator1/1 -> "EKF "/1(x), splitVector/1(x)
  Constant/1 -> Discrete-Time Integrator1/2
  jetIntensityMeasurement/1 -> "EKF "/3(measurement)
  Discrete-Time Integrator2/1 -> "EKF "/4(P)
  Constant1/1 -> Discrete-Time Integrator2/2
  splitVector/1(x1) -> jetIntensityFiltered/1
  splitVector/2(x2) -> jetDerivativeEstimated/1

== system momentumBasedFlight/FLIGHT CONTROLLER (CORE) V3.0/Jets Control/extendedKalmanFilter4jets/EKF_jet3 ==
  input : Inport
  jetIntensityMeasurement : Inport  Port=2
  Constant : Constant  Value=[Config.initT, Config.initTdot]
  Constant1 : Constant  Value=Config.ekf.initP
  Discrete-Time Integrator1 : DiscreteIntegrator  InitialConditionSource=external  SampleTime=Config.tStep  ICPrevOutput=DiscIntNeverNeededParam  ICPrevScaledInput=DiscIntNeverNeededParam
  Discrete-Time Integrator2 : DiscreteIntegrator  InitialConditionSource=external  SampleTime=Config.tStep  ICPrevOutput=DiscIntNeverNeededParam  ICPrevScaledInput=DiscIntNeverNeededParam
  "EKF " : MATLAB Function  TreatAsAtomicUnit=on
  splitVector : MATLAB Function  TreatAsAtomicUnit=on
  jetIntensityFiltered : Outport  VectorParamsAs1DForOutWhenUnconnected=off
  jetDerivativeEstimated : Outport  Port=2  VectorParamsAs1DForOutWhenUnconnected=off
  wires:
  splitVector/2(x2) -> jetDerivativeEstimated/1
  splitVector/1(x1) -> jetIntensityFiltered/1
  Constant1/1 -> Discrete-Time Integrator2/2
  Discrete-Time Integrator2/1 -> "EKF "/4(P)
  jetIntensityMeasurement/1 -> "EKF "/3(measurement)
  Constant/1 -> Discrete-Time Integrator1/2
  Discrete-Time Integrator1/1 -> splitVector/1(x), "EKF "/1(x)
  input/1 -> "EKF "/2(input)
  "EKF "/1(xDot) -> Discrete-Time Integrator1/1
  "EKF "/2(Pdot) -> Discrete-Time Integrator2/1

== system momentumBasedFlight/FLIGHT CONTROLLER (CORE) V3.0/Jets Control/extendedKalmanFilter4jets/EKF_jet4 ==
  input : Inport
  jetIntensityMeasurement : Inport  Port=2
  Constant : Constant  Value=[Config.initT, Config.initTdot]
  Constant1 : Constant  Value=Config.ekf.initP
  Discrete-Time Integrator1 : DiscreteIntegrator  InitialConditionSource=external  SampleTime=Config.tStep  ICPrevOutput=DiscIntNeverNeededParam  ICPrevScaledInput=DiscIntNeverNeededParam
  Discrete-Time Integrator2 : DiscreteIntegrator  InitialConditionSource=external  SampleTime=Config.tStep  ICPrevOutput=DiscIntNeverNeededParam  ICPrevScaledInput=DiscIntNeverNeededParam
  "EKF " : MATLAB Function  TreatAsAtomicUnit=on
  splitVector : MATLAB Function  TreatAsAtomicUnit=on
  jetIntensityFiltered : Outport  VectorParamsAs1DForOutWhenUnconnected=off
  jetDerivativeEstimated : Outport  Port=2  VectorParamsAs1DForOutWhenUnconnected=off
  wires:
  "EKF "/2(Pdot) -> Discrete-Time Integrator2/1
  "EKF "/1(xDot) -> Discrete-Time Integrator1/1
  input/1 -> "EKF "/2(input)
  Discrete-Time Integrator1/1 -> "EKF "/1(x), splitVector/1(x)
  Constant/1 -> Discrete-Time Integrator1/2
  jetIntensityMeasurement/1 -> "EKF "/3(measurement)
  Discrete-Time Integrator2/1 -> "EKF "/4(P)
  Constant1/1 -> Discrete-Time Integrator2/2
  splitVector/1(x1) -> jetIntensityFiltered/1
  splitVector/2(x2) -> jetDerivativeEstimated/1

== system momentumBasedFlight/iRonCub/Forward Dynamics/jetsDyn/Simulink Function ==
  simFunc_getFrameFreeFloatingJacobianJet1Frame : TriggerPort  TriggerType=function-call  IsSimulinkFunction=on  FunctionName=simFunc_getFrameFreeFloatingJacobianJet1Frame  FunctionVisibility=scoped  VariantControl=(inherit)
  Jacobian Left Foot : WBToolboxLibrary/Model/Jacobians/Jacobian  frameName=Frames.JET1_FRAME
      settings: SourceProductName=WholeBodyToolbox
  basePose : ArgIn  DisableCoverage=on  PortDimensions=[4,4]  ArgumentName=basePose
  jointPosition : ArgIn  Port=2  PortDimensions=[robot_config.N_DOF,1]  ArgumentName=jointPosition
  jacobian : ArgOut  DisableCoverage=on  PortDimensions=[6,6+robot_config.N_DOF]  ArgumentName=jacobian
  wires:
  Jacobian Left Foot/1 -> jacobian/1
  jointPosition/1 -> Jacobian Left Foot/2
  basePose/1 -> Jacobian Left Foot/1

== system momentumBasedFlight/iRonCub/Forward Dynamics/jetsDyn/Simulink Function1 ==
  simFunc_getWorldTransformJet2Frame : TriggerPort  TriggerType=function-call  IsSimulinkFunction=on  FunctionName=simFunc_getWorldTransformJet2Frame  FunctionVisibility=scoped  VariantControl=(inherit)
  ForwardKinematics : WBToolboxLibrary/Model/Kinematics/ForwardKinematics  frameName=Frames.JET2_FRAME
      settings: SourceProductName=WholeBodyToolbox
  basePose : ArgIn  DisableCoverage=on  PortDimensions=[4,4]  ArgumentName=basePose
  jointPosition : ArgIn  Port=2  PortDimensions=[robot_config.N_DOF,1]  ArgumentName=jointPosition
  w_H_jet2Frame : ArgOut  DisableCoverage=on  PortDimensions=[4,4]  ArgumentName=w_H_jet2Frame
  wires:
  ForwardKinematics/1 -> w_H_jet2Frame/1
  jointPosition/1 -> ForwardKinematics/2
  basePose/1 -> ForwardKinematics/1
